simulink model "dx_hand_model"  (R2017b)
settings: Solver=ode3  StartTime=0.0  StopTime=inf  FixedStep=0.01  RelTol=1e-3  EnableMultiTasking=on
InitFcn:
  | cutFreq = 0.1; % T
  | sampleTime = 0.01;
  | filt = tf(1,[cutFreq 1]);
  | filt = c2d(filt,sampleTime);
  | 
  | cutFreq2 = 1;
  | filt2 = tf(1,[cutFreq2 1]);
  | filt2 = c2d(filt2,sampleTime);
  | 
  | cutFreq3 = 0.3;
  | filt3 = tf(1,[cutFreq3 1]);
  | filt3 = c2d(filt3,sampleTime);
  | 
  | update_param = 2;
  | 
  | ampliFactor = 1.60;
  | ampliFactorMiddle = 2.00;
  | ampliFactorDistal = 1;
  | 
  | % Set Hand Address
  | % RightHandAddress = '10.100.39.144';
  | RightHandAddress = '10.24.4.91';
  | Verosim = '10.100.39.22'
  | LeftHandAddress = '10.100.39.22'
  | 
  | max_force = 24; % Newton
model workspace (MAT data in the model file):
  SL_ROS_VariableLengthArrays_MaxSizes : struct (value not decoded)
libraries: robotlib x136, simulink_extras x27, simulink x16, etargetslib x2, dspnetwork x2
(part 8 of 19)

== matlab function dx_hand_model/Thumb/Proximal and Distal Phalanx/Mother of Kinematics ==
  data: CMC_AA input; MCP_AA_s output; CMC_FE input; MCP_FE input; l_dist input; l_meta input; xCMC input; yCMC input; zCMC input; xG1 input; yG1 input; zG1 input; xG2 input; yG2 input; zG2 input; xMCP input; yMCP input; zMCP input
function MCP_AA_s = findMCP_AA_fun(CMC_AA,CMC_FE,MCP_FE,l_dist,l_meta,xCMC,yCMC,zCMC,xG1,yG1,zG1,xG2,yG2,zG2,xMCP,yMCP,zMCP)
%unction MCP_AA_s = findMCP_AA_fun(CMC_AA,CMC_FE,MCP_FE,l_dist,l_meta,xCMC,xG1,xG2,xMCP,yCMC,yG1,yG2,yMCP,zCMC,zG1,zG2,zMCP)
%FINDT_FUN
%    T_S = FINDT_FUN(CMC_AA,CMC_FE,MCP_FE,L_DIST,L_META,XCMC,XG1,XG2,XMCP,YCMC,YG1,YG2,YMCP,ZCMC,ZG1,ZG2,ZMCP)

%    This function was generated by the Symbolic Math Toolbox version 8.0.
%    19-Feb-2018 10:44:44

t2 = sin(CMC_FE);
t3 = sin(MCP_FE);
t4 = cos(CMC_AA);
t5 = cos(CMC_FE);
t6 = sin(CMC_AA);
t7 = cos(MCP_FE);
t8 = xCMC.*yG1.*zG2.*1.482138742237647e79;
t9 = xG1.*yG2.*zCMC.*1.482138742237647e79;
t10 = xG2.*yCMC.*zG1.*1.482138742237647e79;
t11 = xCMC.*yMCP.*zG1.*1.482138742237647e79;
t12 = xG1.*yCMC.*zMCP.*1.482138742237647e79;
t13 = xMCP.*yG1.*zCMC.*1.482138742237647e79;
t14 = xCMC.*yG2.*zMCP.*1.482138742237647e79;
t15 = xG2.*yMCP.*zCMC.*1.482138742237647e79;
t16 = xMCP.*yCMC.*zG2.*1.482138742237647e79;
t17 = xG1.*yMCP.*zG2.*1.482138742237647e79;
t18 = xG2.*yG1.*zMCP.*1.482138742237647e79;
t19 = xMCP.*yG2.*zG1.*1.482138742237647e79;
t20 = l_meta.*t2.*xG2.*yG1.*1.482138742237647e79;
t21 = l_meta.*t2.*xG1.*yMCP.*1.482138742237647e79;
t22 = l_meta.*t2.*xMCP.*yG2.*1.482138742237647e79;
t23 = l_meta.*t4.*t5.*yG2.*zG1.*1.482138742237647e79;
t24 = l_meta.*t4.*t5.*yG1.*zMCP.*1.482138742237647e79;
t25 = l_meta.*t4.*t5.*yMCP.*zG2.*1.482138742237647e79;
t26 = l_meta.*t2.*t4.*xG1.*zG2.*9.075482332868094e62;
t27 = l_meta.*t5.*t6.*xG1.*zG2.*1.482138742237647e79;
t28 = l_meta.*t2.*t4.*xMCP.*zG1.*9.075482332868094e62;
t29 = l_meta.*t5.*t6.*xMCP.*zG1.*1.482138742237647e79;
t30 = l_meta.*t2.*t4.*xG2.*zMCP.*9.075482332868094e62;
t31 = l_meta.*t5.*t6.*xG2.*zMCP.*1.482138742237647e79;
t32 = l_dist.*t2.*t7.*xG2.*yG1.*1.482138742237647e79;
t33 = l_dist.*t2.*t7.*xG1.*yMCP.*1.482138742237647e79;
t34 = l_dist.*t2.*t7.*xMCP.*yG2.*1.482138742237647e79;
t35 = l_meta.*t2.*t6.*yG1.*zG2.*9.075482332868094e62;
t36 = l_meta.*t2.*t6.*yMCP.*zG1.*9.075482332868094e62;
t37 = l_meta.*t2.*t6.*yG2.*zMCP.*9.075482332868094e62;
t38 = l_dist.*t4.*t5.*t7.*yG2.*zG1.*1.482138742237647e79;
t39 = l_dist.*t4.*t5.*t7.*yG1.*zMCP.*1.482138742237647e79;
t40 = l_dist.*t4.*t5.*t7.*yMCP.*zG2.*1.482138742237647e79;
t41 = l_dist.*t2.*t4.*t7.*xG1.*zG2.*9.075482332868094e62;
t42 = l_dist.*t5.*t6.*t7.*xG1.*zG2.*1.482138742237647e79;
t43 = l_dist.*t2.*t4.*t7.*xMCP.*zG1.*9.075482332868094e62;
t44 = l_dist.*t5.*t6.*t7.*xMCP.*zG1.*1.482138742237647e79;
t45 = l_dist.*t2.*t4.*t7.*xG2.*zMCP.*9.075482332868094e62;
t46 = l_dist.*t5.*t6.*t7.*xG2.*zMCP.*1.482138742237647e79;
t47 = l_dist.*t2.*t6.*t7.*yG1.*zG2.*9.075482332868094e62;
t48 = l_dist.*t2.*t6.*t7.*yMCP.*zG1.*9.075482332868094e62;
t49 = l_dist.*t2.*t6.*t7.*yG2.*zMCP.*9.075482332868094e62;
t160 = l_dist.*t7.*xG1.*yG2.*1.815096466573619e63;
t161 = l_dist.*t7.*xG2.*yG1.*1.815096466573619e63;
t162 = l_dist.*t7.*xG1.*yMCP.*1.815096466573619e63;
t163 = l_dist.*t7.*xMCP.*yG1.*1.815096466573619e63;
t164 = l_dist.*t7.*xG2.*yMCP.*1.815096466573619e63;
t165 = l_dist.*t7.*xMCP.*yG2.*1.815096466573619e63;
t166 = l_dist.*t5.*t7.*xG1.*yG2.*1.815096466573619e63;
t167 = l_dist.*t5.*t7.*xG2.*yG1.*1.815096466573619e63;
t168 = l_dist.*t5.*t7.*xG1.*yMCP.*1.815096466573619e63;
t169 = l_dist.*t5.*t7.*xMCP.*yG1.*1.815096466573619e63;
t170 = l_dist.*t5.*t7.*xG2.*yMCP.*1.815096466573619e63;
t171 = l_dist.*t5.*t7.*xMCP.*yG2.*1.815096466573619e63;
t172 = l_dist.*t4.*t7.*xG1.*zG2.*2.964277484475295e79;
t173 = l_dist.*t4.*t7.*xG2.*zG1.*2.964277484475295e79;
t174 = l_dist.*t4.*t7.*xG1.*zMCP.*2.964277484475295e79;
t175 = l_dist.*t4.*t7.*xMCP.*zG1.*2.964277484475295e79;
t176 = l_dist.*t4.*t7.*xG2.*zMCP.*2.964277484475295e79;
t177 = l_dist.*t4.*t7.*xMCP.*zG2.*2.964277484475295e79;
t178 = l_dist.*t6.*t7.*yG1.*zG2.*2.964277484475295e79;
t179 = l_dist.*t6.*t7.*yG2.*zG1.*2.964277484475295e79;
t180 = l_dist.*t6.*t7.*yG1.*zMCP.*2.964277484475295e79;
t181 = l_dist.*t6.*t7.*yMCP.*zG1.*2.964277484475295e79;
t182 = l_dist.*t6.*t7.*yG2.*zMCP.*2.964277484475295e79;
t183 = l_dist.*t6.*t7.*yMCP.*zG2.*2.964277484475295e79;
t184 = l_dist.*t2.*t3.*xG1.*yG2.*1.815096466573619e63;
t185 = l_dist.*t2.*t3.*xG2.*yG1.*1.815096466573619e63;
t186 = l_dist.*t2.*t3.*xG1.*yMCP.*1.815096466573619e63;
t187 = l_dist.*t2.*t3.*xMCP.*yG1.*1.815096466573619e63;
t188 = l_dist.*t2.*t3.*xG2.*yMCP.*1.815096466573619e63;
t189 = l_dist.*t2.*t3.*xMCP.*yG2.*1.815096466573619e63;
t190 = l_dist.*t4.*t5.*t7.*xG1.*zG2.*1.111426038966526e47;
t191 = l_dist.*t4.*t5.*t7.*xG2.*zG1.*1.111426038966526e47;
t192 = l_dist.*t4.*t5.*t7.*xG1.*zMCP.*1.111426038966526e47;
t193 = l_dist.*t4.*t5.*t7.*xMCP.*zG1.*1.111426038966526e47;
t194 = l_dist.*t4.*t5.*t7.*xG2.*zMCP.*1.111426038966526e47;
t195 = l_dist.*t4.*t5.*t7.*xMCP.*zG2.*1.111426038966526e47;
t196 = l_dist.*t3.*t4.*t5.*yG1.*zG2.*1.815096466573619e63;
t197 = l_dist.*t2.*t4.*t7.*yG1.*zG2.*1.815096466573619e63;
t198 = l_dist.*t5.*t6.*t7.*yG1.*zG2.*1.111426038966526e47;
t199 = l_dist.*t3.*t4.*t5.*yG2.*zG1.*1.815096466573619e63;
t200 = l_dist.*t2.*t4.*t7.*yG2.*zG1.*1.815096466573619e63;
t201 = l_dist.*t5.*t6.*t7.*yG2.*zG1.*1.111426038966526e47;
t202 = l_dist.*t3.*t4.*t5.*yG1.*zMCP.*1.815096466573619e63;
t203 = l_dist.*t2.*t4.*t7.*yG1.*zMCP.*1.815096466573619e63;
t204 = l_dist.*t5.*t6.*t7.*yG1.*zMCP.*1.111426038966526e47;
t205 = l_dist.*t3.*t4.*t5.*yMCP.*zG1.*1.815096466573619e63;
t206 = l_dist.*t2.*t4.*t7.*yMCP.*zG1.*1.815096466573619e63;
t207 = l_dist.*t5.*t6.*t7.*yMCP.*zG1.*1.111426038966526e47;
t208 = l_dist.*t3.*t4.*t5.*yG2.*zMCP.*1.815096466573619e63;
t209 = l_dist.*t2.*t4.*t7.*yG2.*zMCP.*1.815096466573619e63;
t210 = l_dist.*t5.*t6.*t7.*yG2.*zMCP.*1.111426038966526e47;
t211 = l_dist.*t3.*t4.*t5.*yMCP.*zG2.*1.815096466573619e63;
t212 = l_dist.*t2.*t4.*t7.*yMCP.*zG2.*1.815096466573619e63;
t213 = l_dist.*t5.*t6.*t7.*yMCP.*zG2.*1.111426038966526e47;
t214 = l_dist.*t2.*t3.*t4.*xG1.*zG2.*1.111426038966527e47;
t215 = l_dist.*t3.*t5.*t6.*xG1.*zG2.*1.815096466573619e63;
t216 = l_dist.*t2.*t6.*t7.*xG1.*zG2.*1.815096466573619e63;
t217 = l_dist.*t2.*t3.*t4.*xG2.*zG1.*1.111426038966527e47;
t218 = l_dist.*t3.*t5.*t6.*xG2.*zG1.*1.815096466573619e63;
t219 = l_dist.*t2.*t6.*t7.*xG2.*zG1.*1.815096466573619e63;
t220 = l_dist.*t2.*t3.*t4.*xG1.*zMCP.*1.111426038966527e47;
t221 = l_dist.*t3.*t5.*t6.*xG1.*zMCP.*1.815096466573619e63;
t222 = l_dist.*t2.*t6.*t7.*xG1.*zMCP.*1.815096466573619e63;
t223 = l_dist.*t2.*t3.*t4.*xMCP.*zG1.*1.111426038966527e47;
t224 = l_dist.*t3.*t5.*t6.*xMCP.*zG1.*1.815096466573619e63;
t225 = l_dist.*t2.*t6.*t7.*xMCP.*zG1.*1.815096466573619e63;
t226 = l_dist.*t2.*t3.*t4.*xG2.*zMCP.*1.111426038966527e47;
t227 = l_dist.*t3.*t5.*t6.*xG2.*zMCP.*1.815096466573619e63;
t228 = l_dist.*t2.*t6.*t7.*xG2.*zMCP.*1.815096466573619e63;
t229 = l_dist.*t2.*t3.*t4.*xMCP.*zG2.*1.111426038966527e47;
t230 = l_dist.*t3.*t5.*t6.*xMCP.*zG2.*1.815096466573619e63;
t231 = l_dist.*t2.*t6.*t7.*xMCP.*zG2.*1.815096466573619e63;
t232 = l_dist.*t2.*t3.*t6.*yG1.*zG2.*1.111426038966527e47;
t233 = l_dist.*t2.*t3.*t6.*yG2.*zG1.*1.111426038966527e47;
t234 = l_dist.*t2.*t3.*t6.*yG1.*zMCP.*1.111426038966527e47;
t235 = l_dist.*t2.*t3.*t6.*yMCP.*zG1.*1.111426038966527e47;
t236 = l_dist.*t2.*t3.*t6.*yG2.*zMCP.*1.111426038966527e47;
t237 = l_dist.*t2.*t3.*t6.*yMCP.*zG2.*1.111426038966527e47;
t50 = t160-t161-t162+t163+t164-t165-t166+t167+t168-t169-t170+t171+t172-t173-t174+t175+t176-t177+t178-t179-t180+t181+t182-t183+t184-t185-t186+t187+t188-t189+t190-t191-t192+t193+t194-t195+t196+t197+t198-t199-t200-t201-t202-t203-t204+t205+t206+t207+t208+t209+t210-t211-t212-t213-t214-t215-t216+t217+t218+t219+t220+t221+t222-t223-t224-t225-t226-t227-t228+t229+t230+t231-t232+t233+t234-t235-t236+t237;
t51 = l_dist.*t3.*xG2.*yG1.*1.111426038966526e47;
t52 = l_dist.*t3.*xG1.*yMCP.*1.111426038966526e47;
t53 = l_dist.*t3.*xMCP.*yG2.*1.111426038966526e47;
t54 = l_dist.*t2.*t7.*xG1.*yG2.*1.482138742237647e79;
t55 = l_dist.*t3.*t5.*xG2.*yG1.*1.482138742237647e79;
t56 = l_dist.*t3.*t5.*xG1.*yMCP.*1.482138742237647e79;
t57 = l_dist.*t2.*t7.*xMCP.*yG1.*1.482138742237647e79;
t58 = l_dist.*t2.*t7.*xG2.*yMCP.*1.482138742237647e79;
t59 = l_dist.*t3.*t5.*xMCP.*yG2.*1.482138742237647e79;
t60 = l_dist.*t3.*t4.*xG2.*zG1.*1.815096466573619e63;
t61 = l_dist.*t3.*t4.*xG1.*zMCP.*1.815096466573619e63;
t62 = l_dist.*t3.*t4.*xMCP.*zG2.*1.815096466573619e63;
t63 = l_dist.*t3.*t6.*yG2.*zG1.*1.815096466573619e63;
t64 = l_dist.*t3.*t6.*yG1.*zMCP.*1.815096466573619e63;
t65 = l_dist.*t3.*t6.*yMCP.*zG2.*1.815096466573619e63;
t66 = l_dist.*t4.*t5.*t7.*yG1.*zG2.*1.482138742237647e79;
t67 = l_dist.*t4.*t5.*t7.*yMCP.*zG1.*1.482138742237647e79;
t68 = l_dist.*t4.*t5.*t7.*yG2.*zMCP.*1.482138742237647e79;
t69 = l_dist.*t3.*t4.*t5.*xG1.*zG2.*9.075482332868094e62;
t70 = l_dist.*t2.*t4.*t7.*xG2.*zG1.*9.075482332868094e62;
t71 = l_dist.*t5.*t6.*t7.*xG2.*zG1.*1.482138742237647e79;
t72 = l_dist.*t2.*t4.*t7.*xG1.*zMCP.*9.075482332868094e62;
t73 = l_dist.*t5.*t6.*t7.*xG1.*zMCP.*1.482138742237647e79;
t74 = l_dist.*t3.*t4.*t5.*xMCP.*zG1.*9.075482332868094e62;
t75 = l_dist.*t3.*t4.*t5.*xG2.*zMCP.*9.075482332868094e62;
t76 = l_dist.*t2.*t4.*t7.*xMCP.*zG2.*9.075482332868094e62;
t77 = l_dist.*t5.*t6.*t7.*xMCP.*zG2.*1.482138742237647e79;
t78 = l_dist.*t2.*t3.*t4.*yG1.*zG2.*1.482138742237647e79;
t79 = l_dist.*t3.*t5.*t6.*yG1.*zG2.*9.075482332868094e62;
t80 = l_dist.*t2.*t6.*t7.*yG2.*zG1.*9.075482332868094e62;
t81 = l_dist.*t2.*t6.*t7.*yG1.*zMCP.*9.075482332868094e62;
t82 = l_dist.*t2.*t3.*t4.*yMCP.*zG1.*1.482138742237647e79;
t83 = l_dist.*t3.*t5.*t6.*yMCP.*zG1.*9.075482332868094e62;
t84 = l_dist.*t2.*t3.*t4.*yG2.*zMCP.*1.482138742237647e79;
t85 = l_dist.*t3.*t5.*t6.*yG2.*zMCP.*9.075482332868094e62;
t86 = l_dist.*t2.*t6.*t7.*yMCP.*zG2.*9.075482332868094e62;
t87 = l_dist.*t2.*t3.*t6.*xG2.*zG1.*1.482138742237647e79;
t88 = l_dist.*t2.*t3.*t6.*xG1.*zMCP.*1.482138742237647e79;
t89 = l_dist.*t2.*t3.*t6.*xMCP.*zG2.*1.482138742237647e79;
t91 = xCMC.*yG2.*zG1.*1.482138742237647e79;
t92 = xG1.*yCMC.*zG2.*1.482138742237647e79;
t93 = xG2.*yG1.*zCMC.*1.482138742237647e79;
t94 = xCMC.*yG1.*zMCP.*1.482138742237647e79;
t95 = xG1.*yMCP.*zCMC.*1.482138742237647e79;
t96 = xMCP.*yCMC.*zG1.*1.482138742237647e79;
t97 = xCMC.*yMCP.*zG2.*1.482138742237647e79;
t98 = xG2.*yCMC.*zMCP.*1.482138742237647e79;
t99 = xMCP.*yG2.*zCMC.*1.482138742237647e79;
t100 = xG1.*yG2.*zMCP.*1.482138742237647e79;
t101 = xG2.*yMCP.*zG1.*1.482138742237647e79;
t102 = xMCP.*yG1.*zG2.*1.482138742237647e79;
t103 = l_meta.*t2.*xG1.*yG2.*1.482138742237647e79;
t104 = l_meta.*t2.*xMCP.*yG1.*1.482138742237647e79;
t105 = l_meta.*t2.*xG2.*yMCP.*1.482138742237647e79;
t109 = l_meta.*t4.*t5.*yG1.*zG2.*1.482138742237647e79;
t110 = l_meta.*t4.*t5.*yMCP.*zG1.*1.482138742237647e79;
t111 = l_meta.*t4.*t5.*yG2.*zMCP.*1.482138742237647e79;
t112 = l_meta.*t2.*t4.*xG2.*zG1.*9.075482332868094e62;
t113 = l_meta.*t5.*t6.*xG2.*zG1.*1.482138742237647e79;
t114 = l_meta.*t2.*t4.*xG1.*zMCP.*9.075482332868094e62;
t115 = l_meta.*t5.*t6.*xG1.*zMCP.*1.482138742237647e79;
t116 = l_meta.*t2.*t4.*xMCP.*zG2.*9.075482332868094e62;
t117 = l_meta.*t5.*t6.*xMCP.*zG2.*1.482138742237647e79;
t121 = l_meta.*t2.*t6.*yG2.*zG1.*9.075482332868094e62;
t122 = l_meta.*t2.*t6.*yG1.*zMCP.*9.075482332868094e62;
t123 = l_meta.*t2.*t6.*yMCP.*zG2.*9.075482332868094e62;
t136 = l_dist.*t3.*xG1.*yG2.*1.111426038966526e47;
t137 = l_dist.*t3.*xMCP.*yG1.*1.111426038966526e47;
t138 = l_dist.*t3.*xG2.*yMCP.*1.111426038966526e47;
t139 = l_dist.*t3.*t5.*xG1.*yG2.*1.482138742237647e79;
t140 = l_dist.*t3.*t5.*xMCP.*yG1.*1.482138742237647e79;
t141 = l_dist.*t3.*t5.*xG2.*yMCP.*1.482138742237647e79;
t142 = l_dist.*t3.*t4.*xG1.*zG2.*1.815096466573619e63;
t143 = l_dist.*t3.*t4.*xMCP.*zG1.*1.815096466573619e63;
t144 = l_dist.*t3.*t4.*xG2.*zMCP.*1.815096466573619e63;
t145 = l_dist.*t3.*t6.*yG1.*zG2.*1.815096466573619e63;
t146 = l_dist.*t3.*t6.*yMCP.*zG1.*1.815096466573619e63;
t147 = l_dist.*t3.*t6.*yG2.*zMCP.*1.815096466573619e63;
t148 = l_dist.*t3.*t4.*t5.*xG2.*zG1.*9.075482332868094e62;
t149 = l_dist.*t3.*t4.*t5.*xG1.*zMCP.*9.075482332868094e62;
t150 = l_dist.*t3.*t4.*t5.*xMCP.*zG2.*9.075482332868094e62;
t151 = l_dist.*t2.*t3.*t4.*yG2.*zG1.*1.482138742237647e79;
t152 = l_dist.*t3.*t5.*t6.*yG2.*zG1.*9.075482332868094e62;
t153 = l_dist.*t2.*t3.*t4.*yG1.*zMCP.*1.482138742237647e79;
t154 = l_dist.*t3.*t5.*t6.*yG1.*zMCP.*9.075482332868094e62;
t155 = l_dist.*t2.*t3.*t4.*yMCP.*zG2.*1.482138742237647e79;
t156 = l_dist.*t3.*t5.*t6.*yMCP.*zG2.*9.075482332868094e62;
t157 = l_dist.*t2.*t3.*t6.*xG1.*zG2.*1.482138742237647e79;
t158 = l_dist.*t2.*t3.*t6.*xMCP.*zG1.*1.482138742237647e79;
t159 = l_dist.*t2.*t3.*t6.*xG2.*zMCP.*1.482138742237647e79;
t90 = t8+t9+t10+t11+t12+t13+t14+t15+t16+t17+t18+t19+t20+t21+t22+t23+t24+t25+t26+t27+t28+t29+t30+t31-t32-t33-t34+t35+t36+t37-t38-t39-t40-t41-t42-t43-t44-t45-t46-t47-t48-t49+t51+t52+t53+t54+t55+t56+t57+t58+t59+t60+t61+t62+t63+t64+t65+t66+t67+t68+t69+t70+t71+t72+t73+t74+t75+t76+t77+t78+t79+t80+t81+t82+t83+t84+t85+t86+t87+t88+t89-t91-t92-t93-t94-t95-t96-t97-t98-t99-t100-t101-t102-t103-t104-t105-t109-t110-t111-t112-t113-t114-t115-t116-t117-t121-t122-t123-t136-t137-t138-t139-t140-t141-t142-t143-t144-t145-t146-t147-t148-t149-t150-t151-t152-t153-t154-t155-t156-t157-t158-t159;
t106 = l_dist.*t3.*xG1.*yG2.*2.229194389367849e30;
t107 = l_dist.*t3.*xMCP.*yG1.*2.229194389367849e30;
t108 = l_dist.*t3.*xG2.*yMCP.*2.229194389367849e30;
t118 = l_dist.*t3.*t5.*xG2.*yG1.*1.482138742237647e79;
t119 = l_dist.*t3.*t5.*xG1.*yMCP.*1.482138742237647e79;
t120 = l_dist.*t3.*t5.*xMCP.*yG2.*1.482138742237647e79;
t124 = l_dist.*t3.*t4.*t5.*xG1.*zG2.*9.075482332868094e62;
t125 = l_dist.*t3.*t4.*t5.*xMCP.*zG1.*9.075482332868094e62;
t126 = l_dist.*t3.*t4.*t5.*xG2.*zMCP.*9.075482332868094e62;
t127 = l_dist.*t2.*t3.*t4.*yG1.*zG2.*1.482138742237647e79;
t128 = l_dist.*t3.*t5.*t6.*yG1.*zG2.*9.075482332868094e62;
t129 = l_dist.*t2.*t3.*t4.*yMCP.*zG1.*1.482138742237647e79;
t130 = l_dist.*t3.*t5.*t6.*yMCP.*zG1.*9.075482332868094e62;
t131 = l_dist.*t2.*t3.*t4.*yG2.*zMCP.*1.482138742237647e79;
t132 = l_dist.*t3.*t5.*t6.*yG2.*zMCP.*9.075482332868094e62;
t133 = l_dist.*t2.*t3.*t6.*xG2.*zG1.*1.482138742237647e79;
t134 = l_dist.*t2.*t3.*t6.*xG1.*zMCP.*1.482138742237647e79;
t135 = l_dist.*t2.*t3.*t6.*xMCP.*zG2.*1.482138742237647e79;
t238 = t50.^2;
t239 = t238.*(1.0./4.0);
t240 = l_dist.*t7.*xG2.*yG1.*9.075482332868094e62;
t241 = l_dist.*t7.*xG1.*yMCP.*9.075482332868094e62;
t242 = l_dist.*t7.*xMCP.*yG2.*9.075482332868094e62;
t243 = l_dist.*t5.*t7.*xG1.*yG2.*9.075482332868094e62;
t244 = l_dist.*t5.*t7.*xMCP.*yG1.*9.075482332868094e62;
t245 = l_dist.*t5.*t7.*xG2.*yMCP.*9.075482332868094e62;
t246 = l_dist.*t4.*t7.*xG2.*zG1.*1.482138742237647e79;
t247 = l_dist.*t4.*t7.*xG1.*zMCP.*1.482138742237647e79;
t248 = l_dist.*t4.*t7.*xMCP.*zG2.*1.482138742237647e79;
t249 = l_dist.*t6.*t7.*yG2.*zG1.*1.482138742237647e79;
t250 = l_dist.*t6.*t7.*yG1.*zMCP.*1.482138742237647e79;
t251 = l_dist.*t6.*t7.*yMCP.*zG2.*1.482138742237647e79;
t252 = l_dist.*t2.*t3.*xG2.*yG1.*9.075482332868094e62;
t253 = l_dist.*t2.*t3.*xG1.*yMCP.*9.075482332868094e62;
t254 = l_dist.*t2.*t3.*xMCP.*yG2.*9.075482332868094e62;
t255 = l_dist.*t4.*t5.*t7.*xG2.*zG1.*5.557130194832632e46;
t256 = l_dist.*t4.*t5.*t7.*xG1.*zMCP.*5.557130194832632e46;
t257 = l_dist.*t4.*t5.*t7.*xMCP.*zG2.*5.557130194832632e46;
t258 = l_dist.*t3.*t4.*t5.*yG2.*zG1.*9.075482332868094e62;
t259 = l_dist.*t2.*t4.*t7.*yG2.*zG1.*9.075482332868094e62;
t260 = l_dist.*t5.*t6.*t7.*yG2.*zG1.*5.557130194832632e46;
t261 = l_dist.*t3.*t4.*t5.*yG1.*zMCP.*9.075482332868094e62;
t262 = l_dist.*t2.*t4.*t7.*yG1.*zMCP.*9.075482332868094e62;
t263 = l_dist.*t5.*t6.*t7.*yG1.*zMCP.*5.557130194832632e46;
t264 = l_dist.*t3.*t4.*t5.*yMCP.*zG2.*9.075482332868094e62;
t265 = l_dist.*t2.*t4.*t7.*yMCP.*zG2.*9.075482332868094e62;
t266 = l_dist.*t5.*t6.*t7.*yMCP.*zG2.*5.557130194832632e46;
t267 = l_dist.*t2.*t3.*t4.*xG1.*zG2.*5.557130194832633e46;
t268 = l_dist.*t3.*t5.*t6.*xG1.*zG2.*9.075482332868094e62;
t269 = l_dist.*t2.*t6.*t7.*xG1.*zG2.*9.075482332868094e62;
t270 = l_dist.*t2.*t3.*t4.*xMCP.*zG1.*5.557130194832633e46;
t271 = l_dist.*t3.*t5.*t6.*xMCP.*zG1.*9.075482332868094e62;
t272 = l_dist.*t2.*t6.*t7.*xMCP.*zG1.*9.075482332868094e62;
t273 = l_dist.*t2.*t3.*t4.*xG2.*zMCP.*5.557130194832633e46;
t274 = l_dist.*t3.*t5.*t6.*xG2.*zMCP.*9.075482332868094e62;
t275 = l_dist.*t2.*t6.*t7.*xG2.*zMCP.*9.075482332868094e62;
t276 = l_dist.*t2.*t3.*t6.*yG1.*zG2.*5.557130194832633e46;
t277 = l_dist.*t2.*t3.*t6.*yMCP.*zG1.*5.557130194832633e46;
t278 = l_dist.*t2.*t3.*t6.*yG2.*zMCP.*5.557130194832633e46;
t279 = 1.0./t90;
t_s = [t279.*(t240+t241+t242+t243+t244+t245+t246+t247+t248+t249+t250+t251+t252+t253+t254+t255+t256+t257+t258+t259+t260+t261+t262+t263+t264+t265+t266+t267+t268+t269+t270+t271+t272+t273+t274+t275+t276+t277+t278+my_sqrt(t239-t90.*(t8+t9+t10+t11+t12+t13+t14+t15+t16+t17+t18+t19+t20+t21+t22+t23+t24+t25+t26+t27+t28+t29+t30+t31+t32+t33+t34+t35+t36+t37+t38+t39+t40+t41+t42+t43+t44+t45+t46+t47+t48+t49+t106+t107+t108+t118+t119+t120+t124+t125+t126+t127+t128+t129+t130+t131+t132+t133+t134+t135-xCMC.*yG2.*zG1.*1.482138742237647e79-xG1.*yCMC.*zG2.*1.482138742237647e79-xG2.*yG1.*zCMC.*1.482138742237647e79-xCMC.*yG1.*zMCP.*1.482138742237647e79-xG1.*yMCP.*zCMC.*1.482138742237647e79-xMCP.*yCMC.*zG1.*1.482138742237647e79-xCMC.*yMCP.*zG2.*1.482138742237647e79-xG2.*yCMC.*zMCP.*1.482138742237647e79-xMCP.*yG2.*zCMC.*1.482138742237647e79-xG1.*yG2.*zMCP.*1.482138742237647e79-xG2.*yMCP.*zG1.*1.482138742237647e79-xMCP.*yG1.*zG2.*1.482138742237647e79-l_dist.*t3.*xG2.*yG1.*2.229194389367849e30-l_meta.*t2.*xG1.*yG2.*1.482138742237647e79-l_dist.*t3.*xG1.*yMCP.*2.229194389367849e30-l_dist.*t3.*xMCP.*yG2.*2.229194389367849e30-l_meta.*t2.*xMCP.*yG1.*1.482138742237647e79-l_meta.*t2.*xG2.*yMCP.*1.482138742237647e79-l_dist.*t3.*t5.*xG1.*yG2.*1.482138742237647e79-l_dist.*t2.*t7.*xG1.*yG2.*1.482138742237647e79-l_dist.*t3.*t5.*xMCP.*yG1.*1.482138742237647e79-l_dist.*t2.*t7.*xMCP.*yG1.*1.482138742237647e79-l_dist.*t3.*t5.*xG2.*yMCP.*1.482138742237647e79-l_dist.*t2.*t7.*xG2.*yMCP.*1.482138742237647e79-l_meta.*t2.*t4.*xG2.*zG1.*9.075482332868094e62-l_meta.*t5.*t6.*xG2.*zG1.*1.482138742237647e79-l_meta.*t2.*t4.*xG1.*zMCP.*9.075482332868094e62-l_meta.*t2.*t4.*xMCP.*zG2.*9.075482332868094e62-l_meta.*t5.*t6.*xG1.*zMCP.*1.482138742237647e79-l_meta.*t5.*t6.*xMCP.*zG2.*1.482138742237647e79-l_meta.*t2.*t6.*yG2.*zG1.*9.075482332868094e62-l_meta.*t4.*t5.*yG1.*zG2.*1.482138742237647e79-l_meta.*t2.*t6.*yG1.*zMCP.*9.075482332868094e62-l_meta.*t2.*t6.*yMCP.*zG2.*9.075482332868094e62-l_meta.*t4.*t5.*yMCP.*zG1.*1.482138742237647e79-l_meta.*t4.*t5.*yG2.*zMCP.*1.482138742237647e79-l_dist.*t2.*t3.*t6.*xG1.*zG2.*1.482138742237647e79-l_dist.*t3.*t4.*t5.*xG2.*zG1.*9.075482332868094e62-l_dist.*t2.*t4.*t7.*xG2.*zG1.*9.075482332868094e62-l_dist.*t5.*t6.*t7.*xG2.*zG1.*1.482138742237647e79-l_dist.*t2.*t3.*t6.*xMCP.*zG1.*1.482138742237647e79-l_dist.*t2.*t3.*t6.*xG2.*zMCP.*1.482138742237647e79-l_dist.*t3.*t4.*t5.*xG1.*zMCP.*9.075482332868094e62-l_dist.*t2.*t4.*t7.*xG1.*zMCP.*9.075482332868094e62-l_dist.*t3.*t4.*t5.*xMCP.*zG2.*9.075482332868094e62-l_dist.*t2.*t4.*t7.*xMCP.*zG2.*9.075482332868094e62-l_dist.*t5.*t6.*t7.*xG1.*zMCP.*1.482138742237647e79-l_dist.*t5.*t6.*t7.*xMCP.*zG2.*1.482138742237647e79-l_dist.*t2.*t3.*t4.*yG2.*zG1.*1.482138742237647e79-l_dist.*t3.*t5.*t6.*yG2.*zG1.*9.075482332868094e62-l_dist.*t2.*t6.*t7.*yG2.*zG1.*9.075482332868094e62-l_dist.*t4.*t5.*t7.*yG1.*zG2.*1.482138742237647e79-l_dist.*t2.*t3.*t4.*yG1.*zMCP.*1.482138742237647e79-l_dist.*t2.*t3.*t4.*yMCP.*zG2.*1.482138742237647e79-l_dist.*t3.*t5.*t6.*yG1.*zMCP.*9.075482332868094e62-l_dist.*t2.*t6.*t7.*yG1.*zMCP.*9.075482332868094e62-l_dist.*t3.*t5.*t6.*yMCP.*zG2.*9.075482332868094e62-l_dist.*t2.*t6.*t7.*yMCP.*zG2.*9.075482332868094e62-l_dist.*t4.*t5.*t7.*yMCP.*zG1.*1.482138742237647e79-l_dist.*t4.*t5.*t7.*yG2.*zMCP.*1.482138742237647e79))-l_dist.*t7.*xG1.*yG2.*9.075482332868094e62-l_dist.*t7.*xMCP.*yG1.*9.075482332868094e62-l_dist.*t7.*xG2.*yMCP.*9.075482332868094e62-l_dist.*t2.*t3.*xG1.*yG2.*9.075482332868094e62-l_dist.*t5.*t7.*xG2.*yG1.*9.075482332868094e62-l_dist.*t2.*t3.*xMCP.*yG1.*9.075482332868094e62-l_dist.*t2.*t3.*xG2.*yMCP.*9.075482332868094e62-l_dist.*t5.*t7.*xG1.*yMCP.*9.075482332868094e62-l_dist.*t5.*t7.*xMCP.*yG2.*9.075482332868094e62-l_dist.*t4.*t7.*xG1.*zG2.*1.482138742237647e79-l_dist.*t4.*t7.*xMCP.*zG1.*1.482138742237647e79-l_dist.*t4.*t7.*xG2.*zMCP.*1.482138742237647e79-l_dist.*t6.*t7.*yG1.*zG2.*1.482138742237647e79-l_dist.*t6.*t7.*yMCP.*zG1.*1.482138742237647e79-l_dist.*t6.*t7.*yG2.*zMCP.*1.482138742237647e79-l_dist.*t2.*t3.*t4.*xG2.*zG1.*5.557130194832633e46-l_dist.*t3.*t5.*t6.*xG2.*zG1.*9.075482332868094e62-l_dist.*t2.*t6.*t7.*xG2.*zG1.*9.075482332868094e62-l_dist.*t4.*t5.*t7.*xG1.*zG2.*5.557130194832632e46-l_dist.*t2.*t3.*t4.*xG1.*zMCP.*5.557130194832633e46-l_dist.*t2.*t3.*t4.*xMCP.*zG2.*5.557130194832633e46-l_dist.*t3.*t5.*t6.*xG1.*zMCP.*9.075482332868094e62-l_dist.*t2.*t6.*t7.*xG1.*zMCP.*9.075482332868094e62-l_dist.*t3.*t5.*t6.*xMCP.*zG2.*9.075482332868094e62-l_dist.*t2.*t6.*t7.*xMCP.*zG2.*9.075482332868094e62-l_dist.*t4.*t5.*t7.*xMCP.*zG1.*5.557130194832632e46-l_dist.*t4.*t5.*t7.*xG2.*zMCP.*5.557130194832632e46-l_dist.*t2.*t3.*t6.*yG2.*zG1.*5.557130194832633e46-l_dist.*t3.*t4.*t5.*yG1.*zG2.*9.075482332868094e62-l_dist.*t2.*t4.*t7.*yG1.*zG2.*9.075482332868094e62-l_dist.*t5.*t6.*t7.*yG1.*zG2.*5.557130194832632e46-l_dist.*t2.*t3.*t6.*yG1.*zMCP.*5.557130194832633e46-l_dist.*t2.*t3.*t6.*yMCP.*zG2.*5.557130194832633e46-l_dist.*t3.*t4.*t5.*yMCP.*zG1.*9.075482332868094e62-l_dist.*t2.*t4.*t7.*yMCP.*zG1.*9.075482332868094e62-l_dist.*t3.*t4.*t5.*yG2.*zMCP.*9.075482332868094e62-l_dist.*t2.*t4.*t7.*yG2.*zMCP.*9.075482332868094e62-l_dist.*t5.*t6.*t7.*yMCP.*zG1.*5.557130194832632e46-l_dist.*t5.*t6.*t7.*yG2.*zMCP.*5.557130194832632e46);-t279.*(-t240-t241-t242-t243-t244-t245-t246-t247-t248-t249-t250-t251-t252-t253-t254-t255-t256-t257-t258-t259-t260-t261-t262-t263-t264-t265-t266-t267-t268-t269-t270-t271-t272-t273-t274-t275-t276-t277-t278+my_sqrt(t239-t90.*(t8+t9+t10+t11+t12+t13+t14+t15+t16+t17+t18+t19+t20+t21+t22+t23+t24+t25+t26+t27+t28+t29+t30+t31+t32+t33+t34+t35+t36+t37+t38+t39+t40+t41+t42+t43+t44+t45+t46+t47+t48+t49-t54-t57-t58-t66-t67-t68-t70-t71-t72-t73-t76-t77-t80-t81-t86-t91-t92-t93-t94-t95-t96-t97-t98-t99-t100-t101-t102-t103-t104-t105+t106+t107+t108-t109-t110-t111-t112-t113-t114-t115-t116-t117+t118+t119+t120-t121-t122-t123+t124+t125+t126+t127+t128+t129+t130+t131+t132+t133+t134+t135-l_dist.*t3.*xG2.*yG1.*2.229194389367849e30-l_dist.*t3.*xG1.*yMCP.*2.229194389367849e30-l_dist.*t3.*xMCP.*yG2.*2.229194389367849e30-l_dist.*t3.*t5.*xG1.*yG2.*1.482138742237647e79-l_dist.*t3.*t5.*xMCP.*yG1.*1.482138742237647e79-l_dist.*t3.*t5.*xG2.*yMCP.*1.482138742237647e79-l_dist.*t2.*t3.*t6.*xG1.*zG2.*1.482138742237647e79-l_dist.*t3.*t4.*t5.*xG2.*zG1.*9.075482332868094e62-l_dist.*t2.*t3.*t6.*xMCP.*zG1.*1.482138742237647e79-l_dist.*t2.*t3.*t6.*xG2.*zMCP.*1.482138742237647e79-l_dist.*t3.*t4.*t5.*xG1.*zMCP.*9.075482332868094e62-l_dist.*t3.*t4.*t5.*xMCP.*zG2.*9.075482332868094e62-l_dist.*t2.*t3.*t4.*yG2.*zG1.*1.482138742237647e79-l_dist.*t3.*t5.*t6.*yG2.*zG1.*9.075482332868094e62-l_dist.*t2.*t3.*t4.*yG1.*zMCP.*1.482138742237647e79-l_dist.*t2.*t3.*t4.*yMCP.*zG2.*1.482138742237647e79-l_dist.*t3.*t5.*t6.*yG1.*zMCP.*9.075482332868094e62-l_dist.*t3.*t5.*t6.*yMCP.*zG2.*9.075482332868094e62))+l_dist.*t7.*xG1.*yG2.*9.075482332868094e62+l_dist.*t7.*xMCP.*yG1.*9.075482332868094e62+l_dist.*t7.*xG2.*yMCP.*9.075482332868094e62+l_dist.*t2.*t3.*xG1.*yG2.*9.075482332868094e62+l_dist.*t5.*t7.*xG2.*yG1.*9.075482332868094e62+l_dist.*t2.*t3.*xMCP.*yG1.*9.075482332868094e62+l_dist.*t2.*t3.*xG2.*yMCP.*9.075482332868094e62+l_dist.*t5.*t7.*xG1.*yMCP.*9.075482332868094e62+l_dist.*t5.*t7.*xMCP.*yG2.*9.075482332868094e62+l_dist.*t4.*t7.*xG1.*zG2.*1.482138742237647e79+l_dist.*t4.*t7.*xMCP.*zG1.*1.482138742237647e79+l_dist.*t4.*t7.*xG2.*zMCP.*1.482138742237647e79+l_dist.*t6.*t7.*yG1.*zG2.*1.482138742237647e79+l_dist.*t6.*t7.*yMCP.*zG1.*1.482138742237647e79+l_dist.*t6.*t7.*yG2.*zMCP.*1.482138742237647e79+l_dist.*t2.*t3.*t4.*xG2.*zG1.*5.557130194832633e46+l_dist.*t3.*t5.*t6.*xG2.*zG1.*9.075482332868094e62+l_dist.*t2.*t6.*t7.*xG2.*zG1.*9.075482332868094e62+l_dist.*t4.*t5.*t7.*xG1.*zG2.*5.557130194832632e46+l_dist.*t2.*t3.*t4.*xG1.*zMCP.*5.557130194832633e46+l_dist.*t2.*t3.*t4.*xMCP.*zG2.*5.557130194832633e46+l_dist.*t3.*t5.*t6.*xG1.*zMCP.*9.075482332868094e62+l_dist.*t2.*t6.*t7.*xG1.*zMCP.*9.075482332868094e62+l_dist.*t3.*t5.*t6.*xMCP.*zG2.*9.075482332868094e62+l_dist.*t2.*t6.*t7.*xMCP.*zG2.*9.075482332868094e62+l_dist.*t4.*t5.*t7.*xMCP.*zG1.*5.557130194832632e46+l_dist.*t4.*t5.*t7.*xG2.*zMCP.*5.557130194832632e46+l_dist.*t2.*t3.*t6.*yG2.*zG1.*5.557130194832633e46+l_dist.*t3.*t4.*t5.*yG1.*zG2.*9.075482332868094e62+l_dist.*t2.*t4.*t7.*yG1.*zG2.*9.075482332868094e62+l_dist.*t5.*t6.*t7.*yG1.*zG2.*5.557130194832632e46+l_dist.*t2.*t3.*t6.*yG1.*zMCP.*5.557130194832633e46+l_dist.*t2.*t3.*t6.*yMCP.*zG2.*5.557130194832633e46+l_dist.*t3.*t4.*t5.*yMCP.*zG1.*9.075482332868094e62+l_dist.*t2.*t4.*t7.*yMCP.*zG1.*9.075482332868094e62+l_dist.*t3.*t4.*t5.*yG2.*zMCP.*9.075482332868094e62+l_dist.*t2.*t4.*t7.*yG2.*zMCP.*9.075482332868094e62+l_dist.*t5.*t6.*t7.*yMCP.*zG1.*5.557130194832632e46+l_dist.*t5.*t6.*t7.*yG2.*zMCP.*5.557130194832632e46)];

MCP_AA_s = atan(t_s)*2; 
end
function y = my_sqrt(x)
    y = sqrt(complex(x));
end

== matlab function dx_hand_model/Send to Schunk/Send data to Ros/MATLAB Function - Assign ==
  data: blankMessage input; u input; msg output Bus: SL_Bus_dx_hand_model_sensor_msgs_JointState; timeStamp input; sec input; Nsec input
function msg = assignArray(blankMessage,u,timeStamp,sec,Nsec)
%#codegen

% To set datatype of MSG output:
%  1. Create buses for this model: robotics.ros.createSimulinkBus(gcs)
%  1. Click "Edit Data" in  Toolstrip to open "Ports and Data Manager"
%  2. Select MSG and set datatype to "Bus: SL_Bus_<modelname>_<messageType>"
% See: 
% http://www.mathworks.com/help/simulink/ug/create-structures-in-matlab-function-blocks.html

% blankMessage (sensor_msgs/LaserScan) consists of 
%             Header: [1x1 Header]
%           AngleMin: 0
%           AngleMax: 0
%     AngleIncrement: 0
%      TimeIncrement: 0
%           ScanTime: 0
%           RangeMin: 0
%           RangeMax: 0
%             Ranges: [0x1 single]
%        Intensities: [0x1 single]

% Set Ranges array to have length 10, and modify indices 1, 3, 5 and 7
blankMessage.Header.Seq = timeStamp;
blankMessage.Header.Stamp.Sec = sec;
blankMessage.Header.Stamp.Nsec = Nsec;
blankMessage.Position_SL_Info.CurrentLength = uint32(9); 
blankMessage.Position([1 2 3 4 5 6 7 8 9]) = [u(1) u(2) u(3) u(4) u(5) u(6) u(7) u(8) u(9)];
blankMessage.Velocity_SL_Info.CurrentLength = uint32(9); 
blankMessage.Velocity([1 2 3 4 5 6 7 8 9]) = zeros(1,9);
blankMessage.Effort_SL_Info.CurrentLength = uint32(9); 
blankMessage.Effort([1 2 3 4 5 6 7 8 9]) = zeros(1,9);
%blankMessage.Name.Data_SL_Info.CurrentLength = uint32(9);
%blankMessage.Name.Data([1 2 3 4 5 6 7 8 9]) = ['right_hand_Thumb_Flexion', 'right_hand_Thumb_Opposition', ...
%     'right_hand_Index_Finger_Distal','right_hand_Index_Finger_Proximal','right_hand_Middle_Finger_Distal','right_hand_Middle_Finger_Proximal',...
%     'right_hand_Ring_Finger','right_hand_Pinky','right_hand_index_spread'];

strArrayToAssign = {'right_hand_Thumb_Flexion', 'right_hand_Thumb_Opposition', ...
    'right_hand_Index_Finger_Distal','right_hand_Index_Finger_Proximal','right_hand_Middle_Finger_Distal','right_hand_Middle_Finger_Proximal',...
    'right_hand_Ring_Finger','right_hand_Pinky','right_hand_Finger_Spread'};


% Set the number of strings in the string array.
% msg (sensor_msgs/JointState) includes the following fields
%           Name : array of std_msgs/String (string array)
%   Name_SL_Info : struct with fields CurrentLength, ReceivedLength
numStringsInArray = length(strArrayToAssign);
blankMessage.Name_SL_Info.CurrentLength = uint32(numStringsInArray);

% Set the individual strings in the array
for idx=1:numStringsInArray
    str = strArrayToAssign{idx};
    strLength = length(str);
    blankMessage.Name(idx).Data(1:strLength) = uint8(str);
    blankMessage.Name(idx).Data_SL_Info.CurrentLength = uint32(strLength);
end
msg = blankMessage;

== matlab function dx_hand_model/Index Finger/Pose Generator/Index Direct Kinematics ==
  data: u input; y output; measurements input
function y  = fcn(u, measurements)
%#codegen
xL_mag = measurements(3); % Posizione lungo l'asse x di L rispetto a K [RIMISURA]
offset = measurements(4); % Distanza tra il giunto K e l'appoggio del metacarpo [RIMISURA]
LIIp = measurements(1); % Semispessore del metacarpo e della falange (da tarare)
LJJp = LIIp; % semispessore della falangina (da tarare, non per forza uguale a LIIp)
LLM = measurements(2); % Lunghezza della falange
LAB =  measurements(5);
LBC =  measurements(6);
LCD =  measurements(7);
LDE =  measurements(8);
LEF =  measurements(9);
LBH =  measurements(10); 
LGH =  measurements(11);
LGF =  measurements(12);
LEJ =  measurements(13);
LCI =  measurements(14);
LKB =  measurements(15);
LKNy = measurements(16); %% MISURA
LKNx = measurements(17); %% MISURA
lact = measurements(18); %Lunghezza dell'attuatore. [RIMISURA]
s_slitta = 13.5; % [mm] misurato con il calibro

LA2A1 = 14.36;%13;
LA2B = 16;%16.78;

LKH = LKB + LBH;
LDF = LDE + LEF;
LBD = LBC + LCD;

LKN =  sqrt(LKNx^2 + LKNy^2); %135.6320;
qKN = atan(LKNy / LKNx); %0.1108; % angolo tra il giunto dell'attacco del motore (N) e il giunto K 

xL = -xL_mag; % Derivata  
yL = -(offset); % Distanza tra K e 01

lx = u(1); % Allungamento del motore misurato
qB = u(2); % Angolo inB misurato dal potenziometro (espresso in radianti)

%% Calcolo qK
% Cambiamenti della cinematica del pollice
% il link AB e' diventato la spezzata BA2A1. Tra A2 e A1 c'e' un angolo di
% 115 gradi

% Lunghezza motore piu' spostamento
LA1N = lx + lact;

LA2K = sqrt(LA2B^2 + LKB^2 - 2*LA2B*LKB*cos(qB));

% angolo in A2 del triangolo A2BK
qA2 = my_acos((- LKB^2 + LA2B^2 + LA2K^2)/(2 * LA2B * LA2K));

% NOTA: presente il valore 115, ovvero l'angolo tra A2B e A2A1
LA1K = sqrt(LA2A1^2 + LA2K^2 - 2*LA2A1*LA2K*cos(115 * pi/180 - qA2));

% angolo in N tra A1N e l'orizzontale
qN = my_acos(((- LA1K^2 + LA1N^2 + LKN^2)/(2*LA1N*LKN))) - qKN;

% angolo in K triangolo KBA2
xK1 = ((-LA2B^2 + LA2K^2 + LKB^2)/(2*LA2K*LKB));
qK1 = my_acos(xK1);

% angolo in K triangolo KA1N
xK2 = (-LA1N^2 + LA1K^2 + LKN^2)/(2*LA1K*LKN);
qK2 = my_acos(xK2);

% angolo in K triangolo A2A1K
xK3 = (-LA2A1^2 + LA2K^2 + LA1K^2)/(2*LA2K*LA1K);
qK3 = my_acos(xK3);
        
% Calcolo qK    
qK = pi - (qK1 + qK2 + qK3 + qKN);

%% Calcolo coordinate punti cinematica parallela
% il centro del sistema di riferimento è in K con asse x verso il polso e
% asse y uscente (contratio alle dita)

% punto B
xB = - LKB * cos(qK);  yB = LKB * sin(qK);
% punto H
xH = - LKH * cos(qK);  yH = LKH * sin(qK);
% punto G
xG = xH - LGH*sin(qK);  yG = yH - LGH*cos(qK);
% punto C
xC = xB - LBC*cos(qB - qK); yC = yB - LBC * sin(qB - qK);
% punto D
xD = xC - LCD*cos(qB - qK);   yD = yC - LCD*sin(qB - qK);
% punto I
xI = xC + LCI * sin(qB - qK);   yI = yC - LCI * cos(qB - qK);
% distanza tra L ed I
LLI = sqrt((xI - xL)^2 + (yI - yL)^2);


%% C1: dello slider. Distanza I da L proiettato sullo slider
spessore = LIIp + s_slitta;


% Mine' version
% alpha = atan((yL - yI)/(xL - xI));

% my version
alpha = atan2((yL - yI),(xL - xI))

% Mine Verion
% temp = LLI^2 - spessore^2;
% if (temp < 0)
%    temp = single(0)
% end
% c1 = sqrt(temp);
% 
% % angolo in L del triangolo LIU
% xj1 = (-spessore^2 + LLI^2 + c1^2)/(2*c1*LLI);
% if abs(xj1)>1
%     xj1 = single(1)
% end
% qj1 = abs(my_acos(xj1));

% My version
temp = LLI^2 - spessore^2;

% Vuol dire che ci sono stati errori nella stima dei parametri. La cosa
% migliore \'e considerare l'angolo qj1 uguale a 90° (potrebbe essere pi\'u
% grande

if (temp < 0)
   qj1 = single(pi/2);
   c1 = single(0);
else
    % attenzione: il giunto i potrebbe trovarsi sia a destra che a sinistra
    % del giunto L. Bisogna usare una funzione su 4 quadranti come atan2
    
    % per saperlo devo identificare dove si trova il punto U
    c1 = sqrt(temp);
    xj1 = (-spessore^2 + LLI^2 + c1^2)/(2*c1*LLI);
    qj1 = my_acos(xj1)
end

%% calcolo di qo1

qo1 = qj1 + alpha;
    
%% Calcolo distanze tra punti nella cinematica parallela   
LHD = sqrt((xH - xD)^2 + (yH - yD)^2);
LDG = sqrt((xG - xD)^2 + (yG - yD)^2);


% angolo in G triangolo DGH - puo' diventare ottuso
xG1 = (-LHD^2 + LDG^2 + LGH^2)/(2*LDG*LGH);
if abs(xG1)>1
    xG1=single(1)
end
qG1 = abs(my_acos(xG1));
% angolo in G triangolo FGD - non puo' diventare ottuso
xG2 = (-LDF^2 + LDG^2 + LGF^2)/(2*LDG*LGF);
if abs(xG2)>1
    xG2=single(1)
end

qG2 = abs(my_acos(xG2));
qG = pi - (qG1 + qG2);

%% Seconda falange
% Giunto M del dito
xM = xL - LLM*cos(qo1); yM = yL - LLM*sin(qo1);

% Angolo in D triangolo DGH
xD1 = (-LGH^2 + LHD^2 + LDG^2)/(2*LHD*LDG);
if abs(xD1)>1
    xD1=single(1)
end
qD1 = abs(my_acos(xD1));
% Angolo in D triangolo GFD
xD2 = (-LGF^2 + LDG^2 + LDF^2)/(2*LDG*LDF);
if abs(xD2)>1
    xD2=single(1)
end
qD2 = abs(my_acos(xD2));
% Angolo in D triangolo BDH
xD3 = (-LBH^2 + LHD^2 + LBD^2)/(2*LHD*LBD);
if abs(xD3)>1
    xD3=single(1);
end
qD3 = abs(my_acos(xD3));

qD = pi - (qD1 + qD2 + qD3);

% Giunto E
xE = xD - LDE*cos(qB - qD - qK);
yE = yD - LDE*sin(qB - qD - qK);
% Giunto J
xJ = xE + LEJ*sin(qB - qD - qK);  
yJ = yE - LEJ*cos(qB - qD - qK);
% Distanza JM
LJM = sqrt((xJ - xM)^2 + (yJ - yM)^2);
% calcolo c2
temp = LJM^2 - spessore^2;

% Mine modified version
% if temp < 0
%     temp = single(0);
% end
% c2 = sqrt(temp);
% 
% % Angolo in M triangolo JSM
% xj2 = (-spessore^2 + LJM^2 + c2^2)/(2*c2*LJM);
% if xj2>1
%     xj2=single(1)
% end
% if xj2<-1
%     xj2=single(-1)
% end
% qj2 = my_acos(xj2);

% Antonio Version
% per le considerazioni sugli angoli, vedere il discorso fatto per qj1
if temp < 0
    qj2 = single(pi/2);
    c2 = single(0);
else
    c2 = sqrt(temp);
    xj2 = (-spessore^2 + LJM^2 + c2^2)/(2*c2*LJM);
    qj2 = my_acos(xj2);
end
    
% Antonio Version
qj3 = atan2((yM - yJ),(xM - xJ));
% qj3
% qj2
% % Mine version
% if (xJ - xM)<=0
%     qj3 = atan((yJ - yM)/(xJ - xM));
% else
%     qj3 = pi + atan((yJ - yM)/(xJ - xM))
% end


qo2 = qj2 + qj3 - qo1;

y = [qo1; qo2; qK; qD; qG; qN; c1; c2]
% LIJ = sqrt((xI-xJ)^2 + (yI-yJ)^2);
% LBJ = sqrt((xB-xJ)^2 + (yB-yJ)^2);
% LCL = sqrt((xC-xL)^2 + (yC-yL)^2);
% y = [qo1; qo2; qK; qD; qG; qN; c1; LIJ; LLI];
end

%% my_acos
function y = my_acos(x)
%     if x < 1
%         t = single(1);
%     else
%         if x > 1
%             t = single(1);
%         else
%             t = x;
%         end
%     end
    t = complex(x);
    y = real( acos(t) );
            
end

== matlab function dx_hand_model/Index Finger/Pose Generator/Parameters/Index Parameters ==
  data: y output; x input
function y = fcn(x)

param = zeros(18,1);
param(1) = x(1); % Semispessore del metacarpo e della falange (da tarare)
param(2) = x(2); % Lunghezza della falange
param(3) = x(3); % Posizione lungo l'asse x di L rispetto a K [RIMISURA]
param(4) = x(4); % Distanza tra il giunto K e l'appoggio del metacarpo [RIMISURA
param(5) =  18; % LAB   NOT USED
param(6) =  43; % LBC
param(7) =  9;  % LCD
param(8) =  40; % LDE
param(9) =  27; % LEF
param(10) =  37; % LBH
param(11) =  86; % LGH
param(12) =  46; % LGF
param(13) =  39; % LEJ
param(14) =  14.10; % LCI DIVERSO DA QUELLO MINE'
param(15) =  35; % LKB
% LKN = 144; lunghezza totale
param(16) = 37.75;%LKN*sin(angle);   % LKNy TO CHANGE
param(17) = 140+7.5;%LKN*cos(angle);  % LKNx TO CHANGE
param(18) = 122;%111.5;  % lact
y = param;

== matlab function dx_hand_model/Thumb/Proximal and Distal Phalanx/MATLAB Function2 ==
  data: x output; u input; y output; z output
function [x,y,z] = split(u)

x = u(1);
y = u(2);
z = u(3);

== matlab function dx_hand_model/Thumb/Direct Kinematics/get H/MATLAB Function1 ==
  data: x output; u input; y output; z output
function [x,y,z] = split(u)

x = u(1);
y = u(2);
z = u(3);

== matlab function dx_hand_model/Thumb/Direct Kinematics/get H/MATLAB Function2 ==
  data: x output; u input; y output; z output
function [x,y,z] = split(u)

x = u(1);
y = u(2);
z = u(3);

== matlab function dx_hand_model/Middle Finger/Pose Generator/Parameters/Middle Parameters ==
  data: y output; x input
function y = fcn(x)

param = zeros(18,1);
param(1) = x(1); % Semispessore del metacarpo e della falange (da tarare)
param(2) = x(2); % Lunghezza della falange
param(3) = x(3); % Posizione lungo l'asse x di L rispetto a K [RIMISURA]
param(4) = x(4); % Distanza tra il giunto K e l'appoggio del metacarpo [RIMISURA
param(5) =  18;
param(6) =  41;
param(7) =  9;
param(8) =  52;
param(9) =  21;
param(10) =  37; 
param(11) =  86;
param(12) =  46;
param(13) =  39;
param(14) =  17;
param(15) =  35;
param(16) = 27;
param(17) = 117;
param(18) = 98; %Lunghezza dell'attuatore. [RIMISURA]
y = param;
